simulink library "ESTS_FRIC_HILO"  (R2024b)
settings: Solver=VariableStepAuto  StartTime=0.0  StopTime=10.0  RelTol=1e-3
libraries: ESTS_FRIC_HILO_CONDLOG x1, ESTS_FRIC_HILO_LIM x1, ESTS_FRIC_HILO_PREPROC x1, ESTS_FRIC_HILO_STATE x1
settings Model: Creator=blatak  LastModifiedBy=blatak

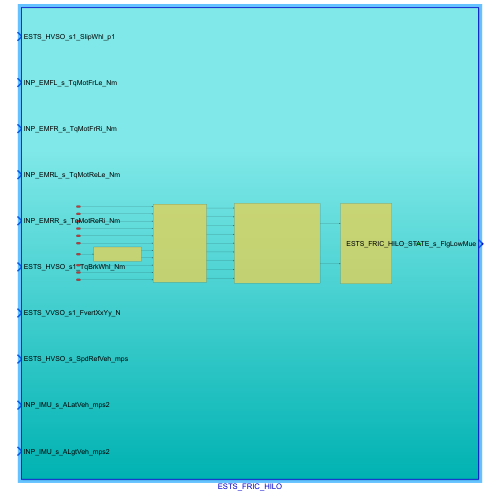
[thumbnail: Simulink's stored preview of the top-level diagram]
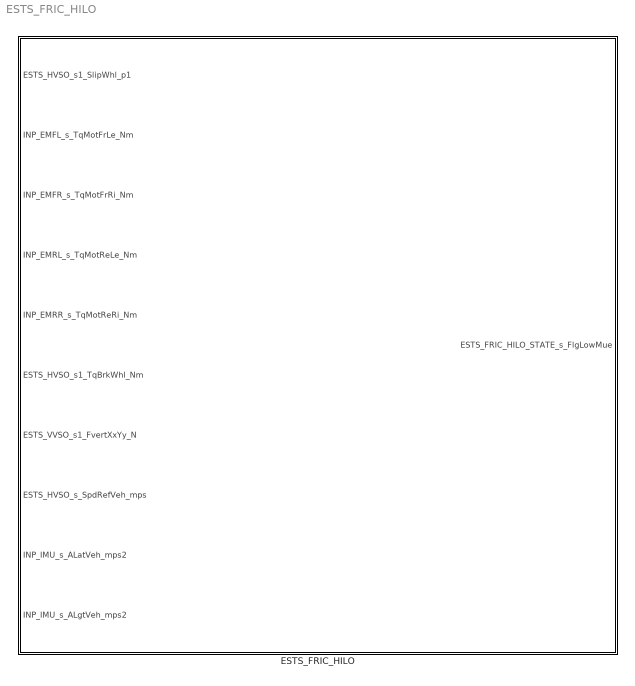
== system ESTS_FRIC_HILO ==
  ESTS_FRIC_HILO : Subsystem

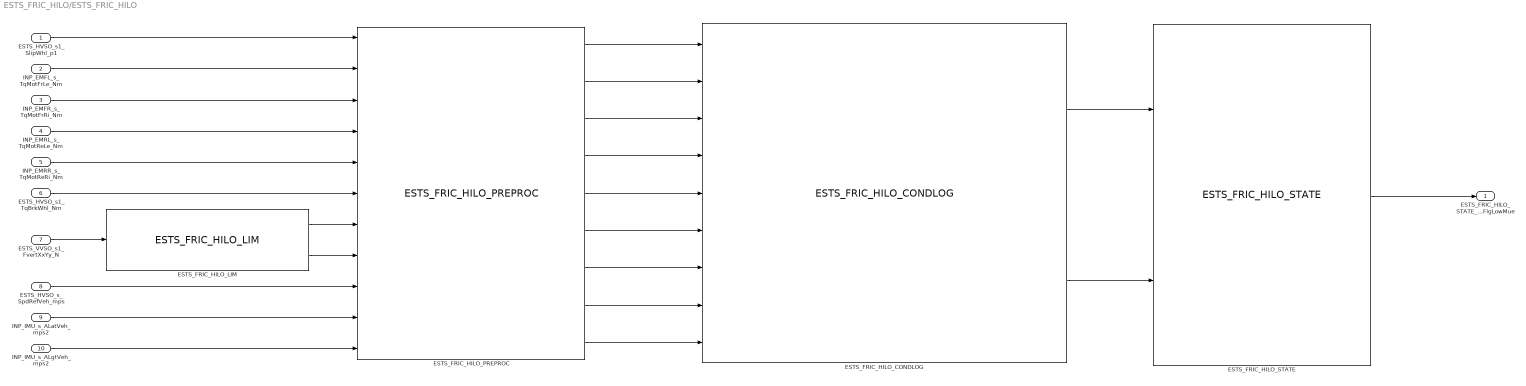
== system ESTS_FRIC_HILO/ESTS_FRIC_HILO ==
  ESTS_HVSO_s1_SlipWhl_p1 : Inport
  INP_EMFL_s_TqMotFrLe_Nm : Inport  Port=2
  INP_EMFR_s_TqMotFrRi_Nm : Inport  Port=3
  INP_EMRL_s_TqMotReLe_Nm : Inport  Port=4
  INP_EMRR_s_TqMotReRi_Nm : Inport  Port=5
  ESTS_HVSO_s1_TqBrkWhl_Nm : Inport  Port=6
  ESTS_VVSO_s1_FvertXxYy_N : Inport  Port=7
  ESTS_HVSO_s_SpdRefVeh_mps : Inport  Port=8
  INP_IMU_s_ALatVeh_mps2 : Inport  Port=9
  INP_IMU_s_ALgtVeh_mps2 : Inport  Port=10
  ESTS_FRIC_HILO_CONDLOG : ESTS_FRIC_HILO_CONDLOG/ESTS_FRIC_HILO_CONDLOG/ESTS_FRIC_HILO_CONDLOG  SystemSampleTime=-1  VariantActivationTime=update diagram  AllowFlexibleInterface=on  Latency=0  AutoFrameSizeCalculation=off
  ESTS_FRIC_HILO_LIM : ESTS_FRIC_HILO_LIM/ESTS_FRIC_HILO_LIM  SystemSampleTime=-1  VariantActivationTime=update diagram  AllowFlexibleInterface=on  Latency=0  AutoFrameSizeCalculation=off
  ESTS_FRIC_HILO_PREPROC : ESTS_FRIC_HILO_PREPROC/ESTS_FRIC_HILO_PREPROC  SystemSampleTime=-1  VariantActivationTime=update diagram  AllowFlexibleInterface=on  Latency=0  AutoFrameSizeCalculation=off
  ESTS_FRIC_HILO_STATE : ESTS_FRIC_HILO_STATE/ESTS_FRIC_HILO_STATE  SystemSampleTime=-1  VariantActivationTime=update diagram  AllowFlexibleInterface=on  Latency=0  AutoFrameSizeCalculation=off
  ESTS_FRIC_HILO_STATE_s_FlgLowMue : Outport
  wires:
  ESTS_FRIC_HILO_PREPROC/2 -> ESTS_FRIC_HILO_CONDLOG/2
  ESTS_FRIC_HILO_PREPROC/9 -> ESTS_FRIC_HILO_CONDLOG/9
  ESTS_FRIC_HILO_CONDLOG/2 -> ESTS_FRIC_HILO_STATE/2
  ESTS_FRIC_HILO_PREPROC/4 -> ESTS_FRIC_HILO_CONDLOG/4
  ESTS_HVSO_s_SpdRefVeh_mps/1 -> ESTS_FRIC_HILO_PREPROC/9
  INP_IMU_s_ALgtVeh_mps2/1 -> ESTS_FRIC_HILO_PREPROC/11
  INP_EMRL_s_TqMotReLe_Nm/1 -> ESTS_FRIC_HILO_PREPROC/4
  ESTS_FRIC_HILO_PREPROC/5 -> ESTS_FRIC_HILO_CONDLOG/5
  INP_IMU_s_ALatVeh_mps2/1 -> ESTS_FRIC_HILO_PREPROC/10
  ESTS_HVSO_s1_SlipWhl_p1/1 -> ESTS_FRIC_HILO_PREPROC/1
  ESTS_FRIC_HILO_PREPROC/6 -> ESTS_FRIC_HILO_CONDLOG/6
  ESTS_VVSO_s1_FvertXxYy_N/1 -> ESTS_FRIC_HILO_LIM/1
  ESTS_FRIC_HILO_PREPROC/3 -> ESTS_FRIC_HILO_CONDLOG/3
  ESTS_FRIC_HILO_CONDLOG/1 -> ESTS_FRIC_HILO_STATE/1
  ESTS_FRIC_HILO_PREPROC/8 -> ESTS_FRIC_HILO_CONDLOG/8
  INP_EMFR_s_TqMotFrRi_Nm/1 -> ESTS_FRIC_HILO_PREPROC/3
  ESTS_FRIC_HILO_PREPROC/7 -> ESTS_FRIC_HILO_CONDLOG/7
  ESTS_FRIC_HILO_PREPROC/1 -> ESTS_FRIC_HILO_CONDLOG/1
  ESTS_FRIC_HILO_STATE/1 -> ESTS_FRIC_HILO_STATE_s_FlgLowMue/1
  INP_EMRR_s_TqMotReRi_Nm/1 -> ESTS_FRIC_HILO_PREPROC/5
  INP_EMFL_s_TqMotFrLe_Nm/1 -> ESTS_FRIC_HILO_PREPROC/2
  ESTS_HVSO_s1_TqBrkWhl_Nm/1 -> ESTS_FRIC_HILO_PREPROC/6
  ESTS_FRIC_HILO_LIM/1 -> ESTS_FRIC_HILO_PREPROC/7
  ESTS_FRIC_HILO_LIM/2 -> ESTS_FRIC_HILO_PREPROC/8
